simulink model "fz8_9"  (R2014a)
settings: Solver=ode45  StartTime=0.0  StopTime=10.0  RelTol=1e-3
values from neighbouring files (symbols this model uses):
  BER = ber(ii)    [eg8_7.m]    (also in eg8_9.m)
undefined symbols (not defined in the file or in its folder): CRC
libraries: commcrc2 x2, commrandsrc2 x1, commchan3 x1, dspmathops x1, commsink2 x1
settings Model: Creator=tzb  LastModifiedBy=tzb

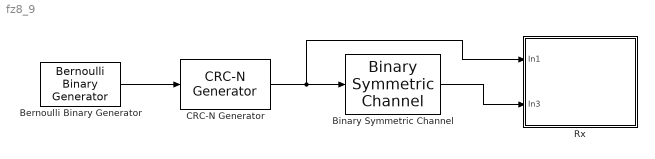
== system fz8_9 ==
  Bernoulli Binary Generator : commrandsrc2/Bernoulli Binary Generator  P=0.5  seed=61  Ts=1/64000000  frameBased=on  sampPerFrame=64  orient=off  outDataType=double
  Binary Symmetric Channel : commchan3/Binary Symmetric Channel  P=BER  s=71  E=off  outDtype=double
  CRC-N Generator : commcrc2/CRC-N Generator  crcMethod=CRC-16  iniStates=[0]  numChecksums=1
  Rx : Subsystem
  wires:
  Bernoulli Binary Generator/1 -> CRC-N Generator/1
  Binary Symmetric Channel/1 -> Rx/2(In3)
  CRC-N Generator/1 -> Rx/1(In1), Binary Symmetric Channel/1

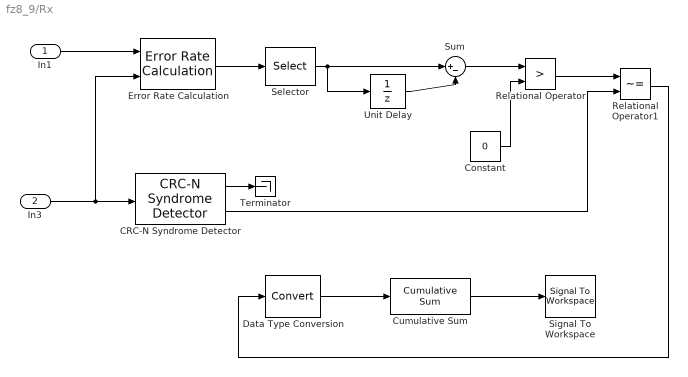
== system fz8_9/Rx ==
  In1 : Inport
  In3 : Inport  Port=2
  CRC-N Syndrome Detector : commcrc2/CRC-N Syndrome Detector  crcMethod=CRC-16  iniStates=[0]  numChecksums=1
  Constant : Constant  Value=0
  Cumulative Sum : dspmathops/Cumulative Sum  dim=Channels (running sum)  InputProcessing=Columns as channels (frame based)  reset_popup=None  outputDataTypeStr=Inherit: Same as accumulator  outputLastDataTypeStr=Inherit: Same as accumulator  outputMin=[]  outputMax=[]  roundingMode=Floor  overflowMode=off
  Data Type Conversion : DataTypeConversion
  Error Rate Calculation : commsink2/Error Rate Calculation  N=0  st_delay=0  cp_mode=Entire frame  subframe=[]  PMode=Port  WsName=ErrorVec  RsMode2=off  stop=off  numErr=100  maxBits=1e6
  Relational Operator : RelationalOperator  Operator=>  OutDataTypeStr=boolean
  Relational Operator1 : RelationalOperator  Operator=~=  OutDataTypeStr=boolean
  Selector : Selector  InputPortWidth=3  Indices=[2]
  Signal To Workspace : SignalToWorkspace  VariableName=MissedFrame
      settings: CopyFcn=dspblkcopystw(gcbh);
  Sum : Sum  Inputs=|+-
  Terminator : Terminator
  Unit Delay : UnitDelay  SampleTime=-1
  wires:
  Data Type Conversion/1 -> Cumulative Sum/1
  Selector/1 -> Unit Delay/1, Sum/1
  Cumulative Sum/1 -> Signal To Workspace/1
  Relational Operator/1 -> Relational Operator1/1
  CRC-N Syndrome Detector/2 -> Relational Operator1/2
  Sum/1 -> Relational Operator/1
  In3/1 -> CRC-N Syndrome Detector/1, Error Rate Calculation/2
  Relational Operator1/1 -> Data Type Conversion/1
  CRC-N Syndrome Detector/1 -> Terminator/1
  Constant/1 -> Relational Operator/2
  Unit Delay/1 -> Sum/2
  In1/1 -> Error Rate Calculation/1
  Error Rate Calculation/1 -> Selector/1
